simulink model "full_diffdrive_ctrl_sim_and_exp_with_arduino"  (R2020a)
settings: Solver=ode3  StartTime=0.0  StopTime=20  FixedStep=0.01  RelTol=1e-3  EnableMultiTasking=on
libraries: xpcobsoletelib x11, simulink x9, arduinolib x4, xpcutilitieslib x3, xpcrtudplib x2, slrtlib x1
(part 2 of 2)

== matlab function full_diffdrive_ctrl_sim_and_exp_with_arduino/To Motor/Motor High Low 1 ==
  data: drivPwmFreq input; genPwmFreq input; d input; H output; L output; A output
function [H,L,A]=fcn(drivPwmFreq,genPwmFreq,d)
%genPwmFreq = fm = 80e6;%refrence
%drivPwmFreq = f = 400;%desire
x = genPwmFreq/drivPwmFreq;
H = d*x;
L = (1-d)*x;
A = 1;

== matlab function full_diffdrive_ctrl_sim_and_exp_with_arduino/To Motor/PWM and Digital Output 5 ==
  data: battVol input; u input; PWM output; DO output
function [PWM, DO]= fcn(battVol,u)   %PWM & D(Digital output) are the output and u is the input (Voltage=24V(because DC motor 24V)).
PWM = abs(u)/battVol;               % PWM equals to value of u (voltage value which was applied)
DO = (sign(u)+1)/2;          % (sign(u): included value of u and its sign)so we will get digital ouput between 0 and 1 (if u = 1 => D = 1 or if u = -1 => D =0)

== matlab function full_diffdrive_ctrl_sim_and_exp_with_arduino/To Motor/Motor High Low 6 ==
  data: drivPwmFreq input; genPwmFreq input; d input; H output; L output; A output
function [H,L,A]=fcn(drivPwmFreq,genPwmFreq,d)
%genPwmFreq = fm = 80e6;%refrence
%drivPwmFreq = f = 400;%desire
x = genPwmFreq/drivPwmFreq;
H = d*x;
L = (1-d)*x;
A = 1;

== matlab function full_diffdrive_ctrl_sim_and_exp_with_arduino/To Motor/PWM and Digital Output 6 ==
  data: battVol input; u input; PWM output; DO output
function [PWM, DO]= fcn(battVol,u)   %PWM & D(Digital output) are the output and u is the input (Voltage=24V(because DC motor 24V)).
PWM = abs(u)/battVol;               % PWM equals to value of u (voltage value which was applied)
DO = (sign(u)+1)/2;          % (sign(u): included value of u and its sign)so we will get digital ouput between 0 and 1 (if u = 1 => D = 1 or if u = -1 => D =0)

== matlab function full_diffdrive_ctrl_sim_and_exp_with_arduino/From Encoder/Convert pulse to rad1 ==
  settings: updateMethod=DISCRETE
  data: u input; ppr input; gearRatio input; outGearBox output
function outGearBox = fcn(u,ppr,gearRatio)

persistent counter_num over_flag
if(isempty(counter_num)), counter_num = 0;end
if(isempty(over_flag)), over_flag = 0;end
pulse2radian = 2*pi/ppr; % 1 pulse = ?? radian

if(double(u) - counter_num > 40000), over_flag = over_flag-1;
elseif(double(u) - counter_num < -40000), over_flag = over_flag+1;
end

inGearBox = (double(u)+over_flag*(2^32 -1))*pulse2radian; 
outGearBox = inGearBox/gearRatio;
counter_num = double(u) ;

== matlab function full_diffdrive_ctrl_sim_and_exp_with_arduino/From Encoder/Convert pulse to rad2 ==
  settings: updateMethod=DISCRETE
  data: u input; ppr input; gearRatio input; outGearBox output
function outGearBox = fcn(u,ppr,gearRatio)

persistent counter_num over_flag
if(isempty(counter_num)), counter_num = 0;end
if(isempty(over_flag)), over_flag = 0;end
pulse2radian = 2*pi/ppr; % 1 pulse = ?? radian

if(double(u) - counter_num > 40000), over_flag = over_flag-1;
elseif(double(u) - counter_num < -40000), over_flag = over_flag+1;
end

inGearBox = (double(u)+over_flag*(2^32 -1))*pulse2radian; 
outGearBox = inGearBox/gearRatio;
counter_num = double(u) ;

== matlab function full_diffdrive_ctrl_sim_and_exp_with_arduino/From Encoder/Convert pulse to rad3 ==
  data: u input; ppr input; gearRatio input; outGearBox output
function outGearBox = fcn(u,ppr,gearRatio)

persistent counter_num over_flag
if(isempty(counter_num)), counter_num = 0;end
if(isempty(over_flag)), over_flag = 0;end
pulse2radian = 2*pi/ppr; % 1 pulse = ?? radian

if(double(u) - counter_num > 40000), over_flag = over_flag-1;
elseif(double(u) - counter_num < -40000), over_flag = over_flag+1;
end

inGearBox = (double(u)+over_flag*(2^32 -1))*pulse2radian; 
outGearBox = inGearBox/gearRatio;
counter_num = double(u) ;

== matlab function full_diffdrive_ctrl_sim_and_exp_with_arduino/From Encoder/Convert pulse to rad4 ==
  data: u input; ppr input; gearRatio input; outGearBox output
function outGearBox = fcn(u,ppr,gearRatio)

persistent counter_num over_flag
if(isempty(counter_num)), counter_num = 0;end
if(isempty(over_flag)), over_flag = 0;end
pulse2radian = 2*pi/ppr; % 1 pulse = ?? radian

if(double(u) - counter_num > 40000), over_flag = over_flag-1;
elseif(double(u) - counter_num < -40000), over_flag = over_flag+1;
end

inGearBox = (double(u)+over_flag*(2^32 -1))*pulse2radian; 
outGearBox = inGearBox/gearRatio;
counter_num = double(u) ;

== matlab function full_diffdrive_ctrl_sim_and_exp_with_arduino/From Encoder/Convert pulse to rad5 ==
  data: u input; ppr input; gearRatio input; outGearBox output
function outGearBox = fcn(u,ppr,gearRatio)

persistent counter_num over_flag
if(isempty(counter_num)), counter_num = 0;end
if(isempty(over_flag)), over_flag = 0;end
pulse2radian = 2*pi/ppr; % 1 pulse = ?? radian

if(double(u) - counter_num > 40000), over_flag = over_flag-1;
elseif(double(u) - counter_num < -40000), over_flag = over_flag+1;
end

inGearBox = (double(u)+over_flag*(2^32 -1))*pulse2radian; 
outGearBox = inGearBox/gearRatio;
counter_num = double(u) ;

== matlab function full_diffdrive_ctrl_sim_and_exp_with_arduino/From Encoder/Convert pulse to rad6 ==
  data: u input; ppr input; gearRatio input; outGearBox output
function outGearBox = fcn(u,ppr,gearRatio)

persistent counter_num over_flag
if(isempty(counter_num)), counter_num = 0;end
if(isempty(over_flag)), over_flag = 0;end
pulse2radian = 2*pi/ppr; % 1 pulse = ?? radian

if(double(u) - counter_num > 40000), over_flag = over_flag-1;
elseif(double(u) - counter_num < -40000), over_flag = over_flag+1;
end

inGearBox = (double(u)+over_flag*(2^32 -1))*pulse2radian; 
outGearBox = inGearBox/gearRatio;
counter_num = double(u) ;

== stateflow chart full_diffdrive_ctrl_sim_and_exp_with_arduino/Manual and auto designer ==
  state Initialization
    entry:
    totalPpr = 14*2*ones(6,1);
    gearRatio = 19.2*3.75*ones(6,1);
    drivPwmFreq = 400; % Hz
    genPwmFreq = 80e6; % Hz
    battVol = 18.4;
    vMax = 2;
    accel = 0.5;
    omegaMax = 1;
    angAccel = 0.3;
    opMode = manual;
    t_dep = [0;0];
    departPose = Xd;
    terminalPose = Xd;
    [isUpdate,Xr] = wayPoints(...
    manual,xytheta,Xd);
    i_max = length(Xr(1,:));
    j_max = i_max;
  state Manual
    entry:
    t_dep = [t;t]; i1 = 1;
    departPose = Xd;
    during:
    [isUpdate,Xr] = wayPoints(manual,xytheta,Xd);
    terminalPose = Xr(:,1);
    if detectChange
    departPose = Xd;
    terminalPose = Xd
    end
  state Semi_autonomous
    entry: [isUpdate,Xr] = wayPoints(manual,xytheta,Xd);
    state Autonomous1
      during:
      if norm(Xr(1:2,i)-Xd(1:2)) < 0.15 && i < i_max
      departPose(1:2) = Xd(1:2);
      terminalPose(1:2) = Xr(1:2,i+1);
      i = i+1;
      t_dep(1) = t;
      end
      if abs(Xr(3,j)-Xd(3)) <  0.05 && j < j_max
      departPose(3) = Xd(3);
      terminalPose(3) = Xr(3,j+1);
      j = j+1;
      t_dep(2) = t;
      end
    state Autonomous
      entry:
      t_dep = [t;t];
      departPose = Xd;
      terminalPose = Xr(:,1);
      i = 1; j = 1;
    (default) -> Autonomous
    Autonomous1 -> Autonomous : [isUpdate]
    Autonomous -> Autonomous1 : [~isUpdate]
  (junction 18) -> (junction 14) : [start && ~manual]
  (default) -> Initialization
  Initialization -> (junction 18) [order 2]
  (junction 14) -> Semi_autonomous
  Initialization -> Manual [order 1] : [manual]
  Manual -> Semi_autonomous : [start && ~manual]
  Semi_autonomous -> Manual : [detectChange]
  data: update function_output; Xp function_output; op function_input; xyo function_input; Xdes function_input; opMode output; totalPpr output; gearRatio output; drivPwmFreq output; genPwmFreq output; battVol output; manual input; xytheta input size=2; detectChange input; t input; start input; Xd_dot input; Xd input; t_dep output; vMax output; accel output; omegaMax output; angAccel output; terminalPose output; departPose output; j_max local; j local; i local; i_max local; i1 local; Xr local size=[3,20]; isUpdate local
  function [update,Xp] = wayPoints(op,xyo,Xdes):
    | function [update,Xp] = wayPoints(op,xyo,Xdes)
    | 
    | persistent X
    | if isempty(X), X = zeros(3,1);end
    | Xp = zeros(3,20);
    |  update = 0;
    | % %Maximum number of column of X is 20
    | 
    | if op
    |     update = 1;
    |     if xyo(1)==2
    |         X(1,1) = 100;
    |     elseif xyo(1)==4
    |         X(1,1) = -100;
    |     elseif xyo(1)==1
    |         X(2,1) = 100;
    |     elseif xyo(1)==3
    |         X(2,1) = -100;
    |     elseif xyo(2)==5
    |         X(3,1) = 100;
    |     elseif xyo(2)==6
    |         X(3,1) = -100;
    |     else
    |         X = Xdes;
    |     end
    | else
    |     X = [
    |     3   6   1                
    |     4   4   2
    |     0   0   0
    |     ];
    | end
    | nPoints = length(X(1,:));
    | Xp(:,1:nPoints) = X;
    | Xp(:,nPoints+1:20) = repmat(X(:,nPoints),1,20-nPoints);

== matlab function full_diffdrive_ctrl_sim_and_exp_with_arduino/Identification/MATLAB Function1 ==
  data: x_hat input; KnTau output
function KnTau = fcn(x_hat)

KnTau = [x_hat(3)/x_hat(2); 1/x_hat(2)];

== matlab function full_diffdrive_ctrl_sim_and_exp_with_arduino/Simulation/Friction ==
  data: w input; vf output
function vf = fcn(w)

vf = 0.13*sigmoidFcn(w);
end

function y = sigmoidFcn(x)
y = 2./(1+exp(-15*x))-1; % element wise computing
end

== matlab function full_diffdrive_ctrl_sim_and_exp_with_arduino/Kinematics for DDMR/controller1 ==
  data: vr input; wd input; Xe input; v output; w output
function [v,w] =  fcn(vr, wd, Xe)      %fcn(Xe)           

% k_rho = 2;
% k_alpha = 1.3;
% rho = sqrt(Xe(1)^2 + Xe(2)^2);
% alpha = Xe(3);
% v = k_rho*rho*cos(alpha);
% w = k_rho*sin(alpha)*cos(alpha) + k_alpha*alpha;
k1 = 3.8;
k2 = 1.8;
k3 = 0.7;

vd = sqrt(vr(1)^2 + vr(2)^2);
v = (vd - k1*abs(vd)*(Xe(1) + Xe(2)*tan(Xe(3))))/cos(Xe(3));
w = wd - (k2*vd*Xe(2) + k3*abs(vd)*tan(Xe(3)))*cos(Xe(3))^2;

== matlab function full_diffdrive_ctrl_sim_and_exp_with_arduino/Kinematics for DDMR/MATLAB Function ==
  data: X_R_dot input; v output; w output
function [v, w] = fcn(X_R_dot)

v = sqrt(X_R_dot(1)^2 + X_R_dot(2)^2);
w = X_R_dot(3);

== matlab function full_diffdrive_ctrl_sim_and_exp_with_arduino/Kinematics for DDMR/es theta calculation ==
  data: es output; dx input; fid output; dy input; fi input
function [es, fid]   = fcn(dx, dy, fi)

fid = atan2(dy,dx);
es = sqrt(dy^2 + dx^2)*cos(fid - fi);

== stateflow chart full_diffdrive_ctrl_sim_and_exp_with_arduino/Identification/Chart2 ==
  state IdentifyKTauFr
    entry:
    %A = [W_ave ones(16,1)];
    %KbRiKtauFr(1:2) = (A'*A)\A'*V;
    %KbRiKtauFr(3) = 1/KbRiKtauFr(1);
    T = 0; t_ref = t; i = 1;
    a_ave = x_hat(2); b_ave = x_hat(3);
    c_ave = x_hat(4);
    during:
    T = t - t_ref; offset = 0;
    Va = (battVol-3 - offset)*sin(2*T)+offset;
    x_hat = UKF(Va,w_measure,dt);
    if T<10*Th
    a_ave = x_hat(2); b_ave = x_hat(3);
    c_ave = x_hat(4);
    else
    a_ave = (a_ave*i + x_hat(2))/(i+1);
    b_ave = (b_ave*i + x_hat(3))/(i+1);
    c_ave = (c_ave*i + x_hat(4))/(i+1);
    i = i+1;
    end
    exit:
    KbRiKtauFr(3) = b_ave/a_ave;
    KbRiKtauFr(4) = 1/a_ave;
    KbRiKtauFr(5) = c_ave/b_ave;
  state Resting
    entry: T = 0; t_ref = t; Va = 0;
    during: T = t - t_ref;
  state Initialization
    entry:
    Va = 2;
    Vinc = 1;
    Th = 1;
    n = 0;
    n_max = 16;
    dt = 0.01;
    w_ave = 0;
    W_ave = zeros(16,1);
    V = W_ave;
    KbRiKtauFr = 0.1*ones(5,1);
    controller = [0;0;0];
    t_contr = 0;
    posError = 0;
    x_hat = 0.1*ones(4,1);
  state VoltageIncrement [commented out]
    entry:
    t_ref = t;
    n = n+1; T = 0;
    if n<n_max/2 + 2
    Va = Va+Vinc;
    else
    Va = Va-Vinc;
    end
    during:
    T = t - t_ref;
  state FeedbackControl
    entry:
    t_ref = t; pos_ref = measuredPos;
    K = KbRiKtauFr(3); tau = KbRiKtauFr(4);
    z = 1.1*a_ave;
    Kd = 1*(2*(tau*z+sqrt(tau*z*(tau*z-1)))-1)/K;
    %Kd=0.45;
    controller(1) = Kd*z; controller(2) = 0;
    controller(3) = Kd;
    during:
    t_contr = t - t_ref;
    posError = desiredPos - ...
    measuredPos + pos_ref;
    Va = PID(posError,controller,battVol,dt) ...
    + desiredVel/K;
    Va = Va+ c_ave/b_ave*sign(desiredVel);
  state AveragingInputOutput [commented out]
    entry:
    i = 1;
    w_ave = w_measure;
    during:
    w_ave = (w_ave*i + w_measure)/(i+1);
    i = i+1; T = t - t_ref;
    exit:
    W_ave(n) = w_ave; V(n) = Va;
  IdentifyKTauFr -> Resting : [T>20*Th]
  Initialization -> IdentifyKTauFr : [1]
  (default) -> Initialization
  Resting -> FeedbackControl : [T>2*Th]
  Initialization -> VoltageIncrement [commented out] : [1]
  VoltageIncrement -> IdentifyKTauFr [commented out] : [n>n_max]
  VoltageIncrement -> AveragingInputOutput [commented out] : [T>Th]
  AveragingInputOutput -> VoltageIncrement [commented out] : [T>2*Th]
  data: err function_input; u function_output; contr function_input; limit function_input; Ts function_input; u_ function_input; y_meas function_input; x function_output; Ts function_input; t_contr output; KbRiKtauFr output size=5; controller output size=3; t input; w_measure input; desiredVel input; desiredPos input; n local; n_max local; Vinc local; Th local; A local size=[16,2]; i local; t_ref local; offset local; a_ave local; b_ave local; measuredPos input; tau local; z local; Kd local; K local; pos_ref local; posError output; x_hat output size=4; T local; dt local; c_ave local; W_ave local size=16; V local size=16; w_ave output; Va output; battVol input
  function u = PID(err,contr,limit,Ts):
    | function u = PID(err,contr,limit,Ts)
    | 
    | persistent integrator;
    | persistent differentiator;
    | persistent err_d1;
    | if isempty(integrator)
    |     integrator = 0;
    |     differentiator = 0;
    |     err_d1 = 0;
    | end
    | tau = 0.04;
    | kp = contr(1); ki = contr(2); kd = contr(3);
    | integrator = integrator + (Ts/2)*(err + err_d1);
    |  % update integrator
    |  differentiator = (2*tau-Ts)/(2*tau+Ts)*differentiator...
    |  + 2/(2*tau+Ts)*(err - err_d1);
    |  % update differentiator
    |  err_d1 = err; % update the err for next time through
    |  % the loop
    |  u = sat(... % implement PID control
    |  kp * err +... % proportional term
    |  ki * integrator +... % integral term
    |  kd * differentiator,... % derivative term
    |  limit... % ensure abs(u)<=limit
    |  );
    |  % implement integrator antiwindup
    |  if ki~=0
    |  u_unsat = kp*err + ki*integrator + kd*differentiator;
    |  integrator = integrator + Ts/ki * (u - u_unsat);
    |  end
    | end
    | function u_sat = sat(value,limit)
    | if value < -limit
    |     u_sat = -limit;
    | elseif value > limit
    |     u_sat = limit;
    | else
    |     u_sat = value;
    | end
    | end
  function x = UKF(u_,y_meas,Ts):
    | function x = UKF(u_,y_meas,Ts)
    | 
    | n = 4;
    | m = 1;
    | Q = 1e-5*diag([1 1000 10000 10000]);
    | R = 1e-2;
    | 
    | nSigma = 2*4+1;
    | 
    | persistent x_ P_ wm W lambda
    | if isempty(x_)
    |     x_= 0.1*ones(4,1); P_ = 1e-1*eye(4);
    |     k=2;
    |     alpha=0.5; beta=1;
    |     lambda=alpha^2*(n+k)-n;
    |     Wm0=lambda/(n+lambda);
    |     Wc0=lambda/((n+lambda)+(1-alpha^2+beta));
    |     Wmi=1/2/(n+lambda);
    |     Wci=Wmi;
    |     wm=Wmi*ones(nSigma,1); wm(1)=Wm0;
    |     W=(eye(nSigma)-wm*ones(1,nSigma))...
    |      *diag([Wc0 Wci*ones(1,2*4)])...
    |      *(eye(nSigma)-wm*ones(1,nSigma))';
    | end
    | 
    | sqrtP = chol(P_,'lower');
    | X_= x_*ones(1,nSigma) + ...
    |         sqrt(n+lambda)*[zeros(4,1) sqrtP -sqrtP];
    | X = X_;
    | for i=1:nSigma
    |     X(:,i)= fd(X_(:,i),u_,Ts);
    | end
    | x1     = X*wm;
    | x = x1(1:4,1);
    | P     = X*W*X'+Q;
    | 
    | %Measurement Update
    | %Re-Generate Sigma Points
    | sqrtP   = chol(P,'lower');
    | X   = x*ones(1,nSigma) + ...
    |         sqrt(n+lambda)*[zeros(4,1) sqrtP -sqrtP];
    | Y   = zeros(m,nSigma);
    | for i=1:nSigma
    |     Y(:,i)= hd(X(:,i));
    | end
    | y   = Y*wm;
    | Pxy = X*W*Y';
    | Pyy = Y*W*Y'+R;
    | KK   = Pxy/Pyy;
    | x_  = x + KK*(y_meas-y);
    | P_  = P - KK*Pyy*KK';
    | 
    | end
    | 
    | function x = fd(x_,u_,Ts)
    | % w_dot = -a*w + b*u - c*sign(w)
    | 
    | % Let x(1)=w, x(2)=a, x(3)=b, x(4)=c, then
    | % x_dot(1) = -x(1)*x(2) + x(3)*u - x(4)*sign(x(1))
    | % x_dot(2) = 0    (since a is constant)
    | % x_dot(3) = 0    (since b is constant)
    | % x_dot(4) = 0    (since c is constant)
    | % In compact form
    | % x_dot = f(x,u)
    | 
    | % Rewritten in discrete form as
    | % x(k) = x(k-1) + f(x(k-1),u(k-1))*Ts
    | 
    | x = x_ + [-x_(1)*x_(2)+x_(3)*u_-x_(4)*sigmoidFcn(x_(1));0;0;0]*Ts;
    | end
    | 
    | function y = hd(x)
    | C = [1 0 0 0];
    | y = C*x;
    | end
    | 
    | function y = sigmoidFcn(x)
    | y = 2/(1+exp(-20*x))-1;
    | end

== matlab function full_diffdrive_ctrl_sim_and_exp_with_arduino/To Motor/Embedded MATLAB Function1 ==
  data: u input; pwm1 output; pwm2 output
function [pwm1,pwm2] = fcn(u)
% This block supports the Embedded MATLAB subset.
% See the help menu for details. 
if u>=1
    u=1;
end
if u<=-1
    u=-1;
end
if u>=0
    pwm1=250*abs(u);
    pwm2=0;
else
    pwm2=250*abs(u);
    pwm1=0;
end

== matlab function full_diffdrive_ctrl_sim_and_exp_with_arduino/To Motor/Embedded MATLAB Function2 ==
  data: u input; pwm1 output; pwm2 output
function [pwm1,pwm2] = fcn(u)
% This block supports the Embedded MATLAB subset.
% See the help menu for details. 
if u>=1
    u=1;
end
if u<=-1
    u=-1;
end
if u>=0
    pwm1=250*abs(u);
    pwm2=0;
else
    pwm2=250*abs(u);
    pwm1=0;
end

== matlab function full_diffdrive_ctrl_sim_and_exp_with_arduino/Kinematics for DDMR/Rotation Matrix (R(fi)) ==
  data: fi input; X_w_dot output; X_R_dot input
function X_w_dot = fcn(fi,X_R_dot)
%#codegen

R = [cos(fi), -sin(fi), 0; sin(fi), cos(fi), 0; 0, 0, 1];
X_w_dot = R*X_R_dot;

== matlab function full_diffdrive_ctrl_sim_and_exp_with_arduino/Kinematics for DDMR/Trajectory velocity generation1 ==
  data: t input; X_r_dot output; t_dep input; Vmax input; accel input; omegaMax input; angAccel input; terminalPose input; departPose input
function X_r_dot = fcn(t,t_dep,Vmax,accel,omegaMax,angAccel,terminalPose,departPose)
%#codegen

Vmax = abs(Vmax); omegaMax = abs(omegaMax);
if Vmax == 0
    Vmax = 1e-5;
end
if omegaMax ==0
    omegaMax = 1e-5;
end
% Vmax = 4; % maximum velocity
%accel = 0.5;      % acceleration
% omegaMax = 3;
%angAccel = 0.7;

X_r_dot = zeros(3,1);


dX = terminalPose(1:2)-departPose(1:2);
norm_dX = norm(dX);
two_rmin = Vmax^2/accel;
dtheta = terminalPose(3)-departPose(3);
norm_dtheta = abs(dtheta);
two_thetamin = omegaMax^2/angAccel;

if norm_dX > two_rmin
    ta = Vmax/accel;                   % acceleration period
    tad = (norm_dX-two_rmin)/Vmax; % acc to deceleration period
    td = ta + tad;                  % start deceleration
    te = ta + td;                   % end deceleration
    if (t-t_dep(1)) < ta
        speed = accel*(t-t_dep(1));
    elseif ta <= (t-t_dep(1)) && (t-t_dep(1)) < td
        speed = Vmax;
    elseif td <= (t-t_dep(1)) && (t-t_dep(1)) < te
        speed = -accel*(t-t_dep(1)-td) + Vmax;
    else
        speed = 0;
    end
else
    tp = sqrt(norm_dX/accel);
    te = 2*tp;
    Vp = accel*tp;
    if (t-t_dep(1)) < tp
        speed = accel*(t-t_dep(1));
    elseif tp <= (t-t_dep(1)) && (t-t_dep(1)) < te
        speed = -accel*(t-t_dep(1)-tp)+Vp;
    else
        speed = 0;
    end
end
if norm_dX~=0
    X_r_dot(1:2) = speed*dX/norm_dX;
end

if norm_dtheta > two_thetamin
    ta = omegaMax/angAccel;                   % acceleration period
    tad = (norm_dtheta-two_thetamin)/omegaMax; % acc to deceleration period
    td = ta + tad;                  % start deceleration
    te = ta + td;                   % end deceleration
    if (t-t_dep(2)) < ta
        omegaSpeed = angAccel*(t-t_dep(2));
    elseif ta <= (t-t_dep(2)) && (t-t_dep(2)) < td
        omegaSpeed = omegaMax;
    elseif td <= (t-t_dep(2)) && (t-t_dep(2)) < te
        omegaSpeed = -angAccel*(t-t_dep(2)-td) + omegaMax;
    else
        omegaSpeed = 0;
    end
else
    tp = sqrt(norm_dtheta/angAccel);
    te = 2*tp;
    omegap = angAccel*tp;
    if (t-t_dep(2)) < tp
        omegaSpeed = angAccel*(t-t_dep(2));
    elseif tp <= (t-t_dep(2)) && (t-t_dep(2)) < te
        omegaSpeed = -angAccel*(t-t_dep(2)-tp)+omegap;
    else
        omegaSpeed = 0;
    end
end
X_r_dot(3) = omegaSpeed*sign(dtheta);

== matlab function full_diffdrive_ctrl_sim_and_exp_with_arduino/Kinematics for DDMR/forward kinematic ==
  data: fi input; fi_R_dot input; X_R_dot output; fi_L_dot input
function X_R_dot = M_inv(fi,fi_R_dot, fi_L_dot)
r = 0.07;      %wheel radius
b = 0.22; 

v = r*[0.5 0.5]*[fi_R_dot; fi_L_dot];
w = r*[0.5/b -0.5/b]*[fi_R_dot; fi_L_dot];
X_R_dot = [cos(fi) 0;sin(fi) 0; 0 1]*[v; w];

== matlab function full_diffdrive_ctrl_sim_and_exp_with_arduino/Kinematics for DDMR/invers Rotation Matrix (R(fi)) ==
  data: fi input; X_R output; X_w input
function X_R = fcn(fi,X_w)
%#codegen

R = [cos(fi), sin(fi), 0; -sin(fi), cos(fi), 0; 0, 0, 1];
X_R = R*X_w;

== matlab function full_diffdrive_ctrl_sim_and_exp_with_arduino/Kinematics for DDMR/invers kinematic ==
  data: v input; fi_R_dot output; w input; fi_L_dot output
function [fi_R_dot, fi_L_dot] = M_inv(v, w)
r = 0.07;      %wheel radius
b = 0.22; 
fi_R_dot = (v + w*b)/r;
fi_L_dot = (v - w*b)/r;

== matlab function full_diffdrive_ctrl_sim_and_exp_with_arduino/To Motor/Motor High Low 2 ==
  data: drivPwmFreq input; genPwmFreq input; d input; H output; L output; A output
function [H,L,A]=fcn(drivPwmFreq,genPwmFreq,d)
%genPwmFreq = fm = 80e6;%refrence
%drivPwmFreq = f = 400;%desire
x = genPwmFreq/drivPwmFreq;
H = d*x;
L = (1-d)*x;
A = 1;

== matlab function full_diffdrive_ctrl_sim_and_exp_with_arduino/To Motor/PWM and Digital Output 2 ==
  data: battVol input; u input; PWM output; DO output
function [PWM, DO]= fcn(battVol,u)   %PWM & D(Digital output) are the output and u is the input (Voltage=24V(because DC motor 24V)).
PWM = abs(u)/battVol;               % PWM equals to value of u (voltage value which was applied)
DO = (sign(u)+1)/2;          % (sign(u): included value of u and its sign)so we will get digital ouput between 0 and 1 (if u = 1 => D = 1 or if u = -1 => D =0)

== matlab function full_diffdrive_ctrl_sim_and_exp_with_arduino/To Motor/Motor High Low 3 ==
  data: drivPwmFreq input; genPwmFreq input; d input; H output; L output; A output
function [H,L,A]=fcn(drivPwmFreq,genPwmFreq,d)
%genPwmFreq = fm = 80e6;%refrence
%drivPwmFreq = f = 400;%desire
x = genPwmFreq/drivPwmFreq;
H = d*x;
L = (1-d)*x;
A = 1;
